simulink model "legacy_torque_controller"  (R2015a)
settings: Solver=ode45  StartTime=0.0  StopTime=10.0  RelTol=1e-3
undefined symbols (not defined in the file): A1_notch_f1, A2_notch_f1, B1_notch_f1, B2_notch_f1, gain_nodes_sea_torque, j_motor, K_notch_f1, k_sea_low, karnopp_model_coulomb_friction, karnopp_model_recursive_filter_sample_number, karnopp_model_static_friction, karnopp_model_velocity_deadzone, kd_sea_percent_of_critical_damping, kp_sea_torque, lateral_motor_efficiency, LEG_MTR_GEAR_RATIO, loaded_unloaded_torque_threshold, max_sagittal_loaded_torque, max_sagittal_unloaded_torque, motor_efficiency_compensation, sample_time, sea_control_torque_cmd_small_threshold
libraries: simulink x4, dsparch4 x1
settings Model: Creator=wmartin  LastModifiedBy=wmartin

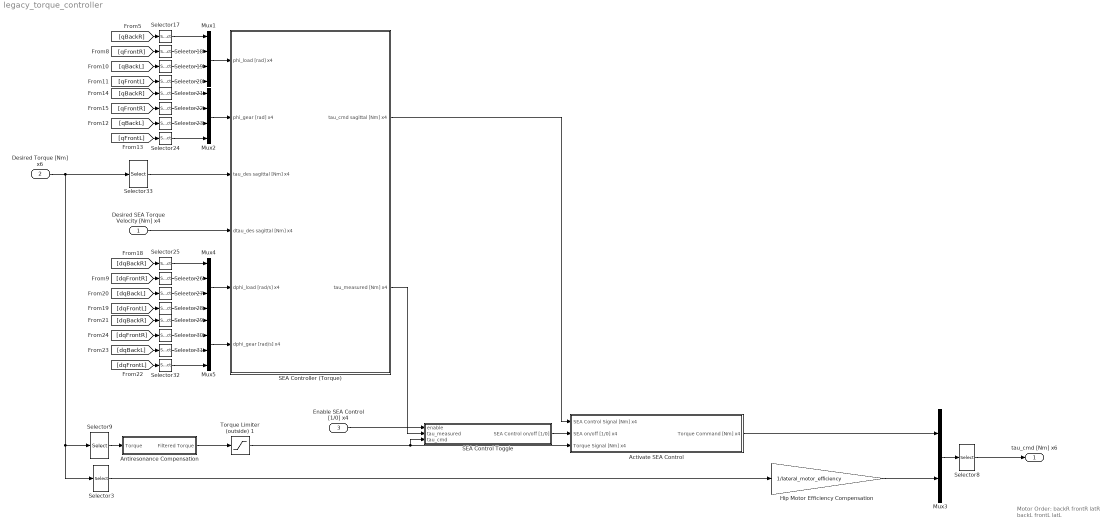
== system legacy_torque_controller ==
  note: Motor Order:
      |
      | backR
      | frontR
      | latR
      | backL
      | frontL
      | latL
  Desired SEA Torque Velocity [Nm] x4 : Inport  OutDataTypeStr=double  PortDimensions=4  SampleTime=sample_time
  Desired Torque [Nm] x6 : Inport  Port=2  OutDataTypeStr=double  PortDimensions=6  SampleTime=sample_time
  Enable SEA Control [1/0] x4 : Inport  Port=3  OutDataTypeStr=boolean  PortDimensions=4  SampleTime=sample_time
  Activate SEA Control : Subsystem
  Antiresonance Compensation : Subsystem
  Hip Motor Efficiency Compensation : Gain  Gain=1/lateral_motor_efficiency
  Mux{1..2,4..5} (4 alike) : Mux
  Mux3 : Mux  Inputs=2
  SEA Control Toggle : Subsystem
  SEA Controller (Torque) : Subsystem
  Selector{17..20,25..28} (8 alike) : Selector  InputPortWidth=2  Indices=[1]
  Selector{21..24,29..32} (8 alike) : Selector  InputPortWidth=2  Indices=[2]
  Selector3 : Selector  InputPortWidth=6  Indices=[3 6]
  Selector33 : Selector  InputPortWidth=6  Indices=[1 2 4 5]
  Selector8 : Selector  InputPortWidth=6  Indices=[1 2 5 3 4 6]
  Selector9 : Selector  InputPortWidth=6  Indices=[1 2 4 5]
  Torque Limiter (outside) 1 : Saturate  UpperLimit=max_sagittal_unloaded_torque  LowerLimit=-max_sagittal_unloaded_torque
      settings: AttributesFormatString=Hi: %<UpperLimit>\nLo: %<LowerLimit>
  tau_cmd [Nm] x6 : Outport  OutDataTypeStr=double  PortDimensions=6  SampleTime=0  InitialOutput=[0 0 0 0 0 0]
  wires:
  Desired Torque [Nm] x6/1 -> Selector9/1, Selector3/1, Selector33/1
  Mux1/1 -> SEA Controller (Torque)/1(phi_load [rad] x4)
  [qBackR] -> Selector17/1
  Selector17/1 -> Mux1/1
  Selector19/1 -> Mux1/3
  Selector18/1 -> Mux1/2
  Selector20/1 -> Mux1/4
  [qFrontR] -> Selector18/1
  [qBackL] -> Selector19/1
  [qFrontL] -> Selector20/1
  Mux2/1 -> SEA Controller (Torque)/2(phi_gear [rad] x4)
  [qBackR] -> Selector21/1
  Selector21/1 -> Mux2/1
  Selector23/1 -> Mux2/3
  Selector22/1 -> Mux2/2
  Selector24/1 -> Mux2/4
  [qFrontR] -> Selector22/1
  [qBackL] -> Selector23/1
  [qFrontL] -> Selector24/1
  Mux4/1 -> SEA Controller (Torque)/5(dphi_load [rad/s] x4)
  [dqBackR] -> Selector25/1
  Selector25/1 -> Mux4/1
  Selector27/1 -> Mux4/3
  Selector26/1 -> Mux4/2
  Selector28/1 -> Mux4/4
  [dqFrontR] -> Selector26/1
  [dqBackL] -> Selector27/1
  [dqFrontL] -> Selector28/1
  Mux5/1 -> SEA Controller (Torque)/6(dphi_gear [rad/s] x4)
  [dqBackR] -> Selector29/1
  Selector29/1 -> Mux5/1
  Selector31/1 -> Mux5/3
  Selector30/1 -> Mux5/2
  Selector32/1 -> Mux5/4
  [dqFrontR] -> Selector30/1
  [dqBackL] -> Selector31/1
  [dqFrontL] -> Selector32/1
  Selector33/1 -> SEA Controller (Torque)/3(tau_des sagittal [Nm] x4)
  Desired SEA Torque Velocity [Nm] x4/1 -> SEA Controller (Torque)/4(dtau_des sagittal [Nm] x4)
  Selector9/1 -> Antiresonance Compensation/1(Torque)
  SEA Controller (Torque)/2(tau_measured [Nm] x4) -> SEA Control Toggle/2(tau_measured)
  Torque Limiter (outside) 1/1 -> SEA Control Toggle/3(tau_cmd), Activate SEA Control/3(Torque Signal [Nm] x4)
  Selector8/1 -> tau_cmd [Nm] x6/1
  Selector3/1 -> Hip Motor Efficiency Compensation/1
  Mux3/1 -> Selector8/1
  Enable SEA Control [1/0] x4/1 -> SEA Control Toggle/1(enable)
  Antiresonance Compensation/1(Filtered Torque) -> Torque Limiter (outside) 1/1
  Activate SEA Control/1(Torque Command [Nm] x4) -> Mux3/1
  Hip Motor Efficiency Compensation/1 -> Mux3/2
  SEA Control Toggle/1(SEA Control on/off [1/0]) -> Activate SEA Control/2("SEA on/off [1/0] x4 ")
  SEA Controller (Torque)/1(tau_cmd sagittal [Nm] x4) -> Activate SEA Control/1(SEA Control Signal [Nm] x4)

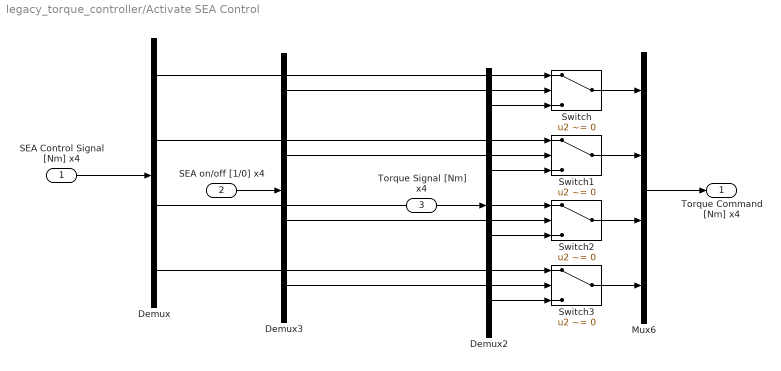
== system legacy_torque_controller/Activate SEA Control ==
  SEA Control Signal [Nm] x4 : Inport
  "SEA on/off [1/0] x4 " : Inport  Port=2
  Torque Signal [Nm] x4 : Inport  Port=3
  Demux : Demux
  Demux2 : Demux
  Demux3 : Demux
  Mux6 : Mux
  Switch{,1..3} (4 alike) : Switch  Criteria=u2 ~= 0
  Torque Command [Nm] x4 : Outport
  wires:
  Torque Signal [Nm] x4/1 -> Demux2/1
  "SEA on/off [1/0] x4 "/1 -> Demux3/1
  SEA Control Signal [Nm] x4/1 -> Demux/1
  Demux2/3 -> Switch2/3
  Demux/2 -> Switch1/1
  Demux3/4 -> Switch3/2
  Demux2/4 -> Switch3/3
  Demux/4 -> Switch3/1
  Switch2/1 -> Mux6/3
  Demux/3 -> Switch2/1
  Demux3/2 -> Switch1/2
  Demux3/3 -> Switch2/2
  Mux6/1 -> Torque Command [Nm] x4/1
  Demux3/1 -> Switch/2
  Switch3/1 -> Mux6/4
  Switch1/1 -> Mux6/2
  Switch/1 -> Mux6/1
  Demux/1 -> Switch/1
  Demux2/1 -> Switch/3
  Demux2/2 -> Switch1/3

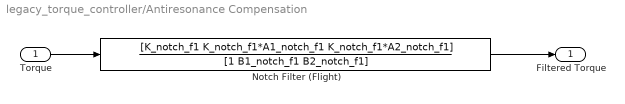
== system legacy_torque_controller/Antiresonance Compensation ==
  Torque : Inport
  Notch Filter (Flight) : DiscreteTransferFcn  Numerator=[K_notch_f1 K_notch_f1*A1_notch_f1 K_notch_f1*A2_notch_f1]  Denominator=[1 B1_notch_f1 B2_notch_f1]  SampleTime=sample_time
  Filtered Torque : Outport
  wires:
  Notch Filter (Flight)/1 -> Filtered Torque/1
  Torque/1 -> Notch Filter (Flight)/1

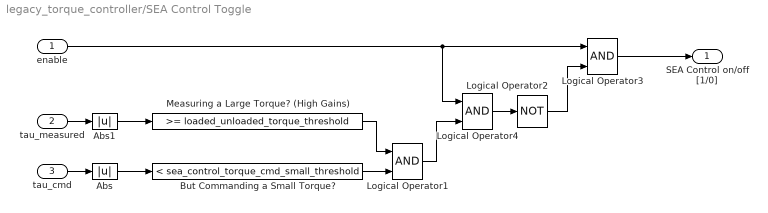
== system legacy_torque_controller/SEA Control Toggle ==
  enable : Inport
  tau_measured : Inport  Port=2
  tau_cmd : Inport  Port=3
  Abs : Abs
  Abs1 : Abs
  But Commanding a Small Torque? : simulink/Logic and Bit Operations/Compare To Constant  relop=<  const=sea_control_torque_cmd_small_threshold  OutDataTypeStr=boolean
  Logical Operator1 : Logic  AllPortsSameDT=off  OutDataTypeStr=boolean
  Logical Operator2 : Logic  Operator=NOT  AllPortsSameDT=off  OutDataTypeStr=boolean
  Logical Operator3 : Logic  AllPortsSameDT=off  OutDataTypeStr=boolean
  Logical Operator4 : Logic  AllPortsSameDT=off  OutDataTypeStr=boolean
  Measuring a Large Torque? (High Gains) : simulink/Logic and Bit Operations/Compare To Constant  relop=>=  const=loaded_unloaded_torque_threshold  OutDataTypeStr=boolean
  SEA Control on/off [1/0] : Outport
  wires:
  Measuring a Large Torque? (High Gains)/1 -> Logical Operator1/1
  enable/1 -> Logical Operator3/1, Logical Operator4/1
  Logical Operator4/1 -> Logical Operator2/1
  Logical Operator2/1 -> Logical Operator3/2
  Logical Operator3/1 -> SEA Control on/off [1/0]/1
  Abs1/1 -> Measuring a Large Torque? (High Gains)/1
  tau_measured/1 -> Abs1/1
  Abs/1 -> But Commanding a Small Torque?/1
  tau_cmd/1 -> Abs/1
  Logical Operator1/1 -> Logical Operator4/2
  But Commanding a Small Torque?/1 -> Logical Operator1/2

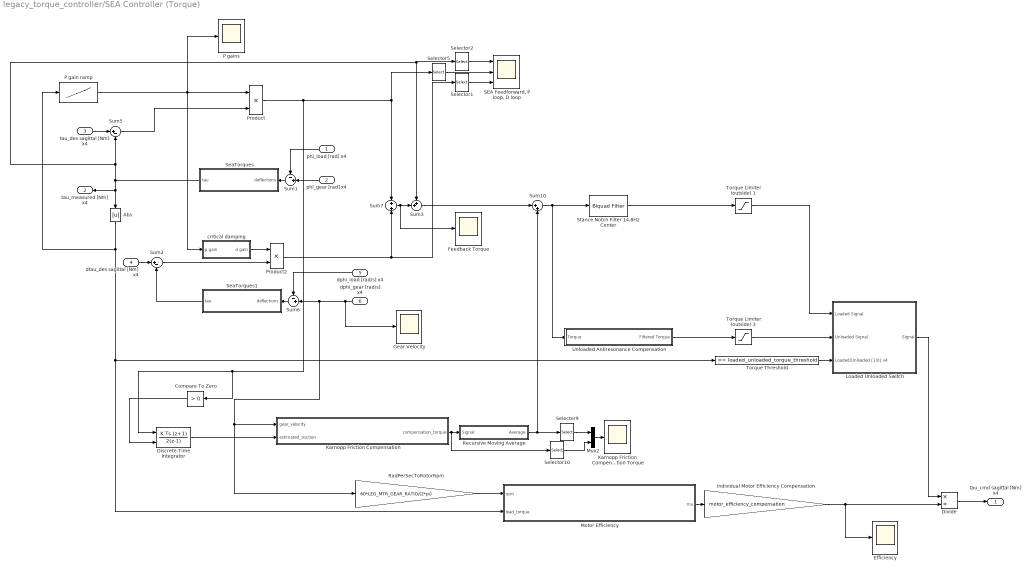
== system legacy_torque_controller/SEA Controller (Torque) ==
  phi_load [rad] x4 : Inport
  phi_gear [rad] x4 : Inport  Port=2
  tau_des sagittal [Nm] x4 : Inport  Port=3
  dtau_des sagittal [Nm] x4 : Inport  Port=4
  dphi_load [rad/s] x4 : Inport  Port=5
  dphi_gear [rad/s] x4 : Inport  Port=6
  Abs : Abs
  Compare To Zero : simulink/Logic and Bit Operations/Compare To Zero  relop=>  OutDataTypeStr=boolean
  Discrete-Time Integrator : DiscreteIntegrator  IntegratorMethod=Integration: Trapezoidal  gainval=karnopp_model_integration_constant  ExternalReset=either  InitialConditionSetting=State (most efficient)  SampleTime=sample_time  LimitOutput=on  UpperSaturationLimit=karnopp_model_static_friction  LowerSaturationLimit=-karnopp_model_static_friction
  Divide : Product  Inputs=*/
  Efficiency : Scope
      settings: YMin=0.45  YMax=0.775  SaveName=ScopeData4  SampleInput=on
  Feedback Torque : Scope
      settings: YMin=-150  YMax=125  SaveName=ScopeData9  SampleInput=on
  Gear Velocity : Scope
      settings: YMin=-0.25  YMax=0.3  SaveName=ScopeData8  SampleInput=on
  Individual Motor Efficiency Compensation : Gain  Gain=motor_efficiency_compensation
  Karnopp Friction Compensation : MATLAB Function  TreatAsAtomicUnit=on
  Karnopp Friction Compensation Torque : Scope
      settings: YMin=-40  YMax=40  SaveName=ScopeData10  SampleInput=on
  Loaded Unloaded Switch : Subsystem
  Motor Efficiency : MATLAB Function  TreatAsAtomicUnit=on
  Mux2 : Mux  Inputs=2
  P gain ramp : Lookup_n-D  NumberOfTableDimensions=1  BreakpointsForDimension1=gain_nodes_sea_torque  Table=kp_sea_torque  InternalRulePriority=Speed  RndMeth=Simplest  InputSameDT=on
  P gains : Scope
      settings: YMin=0.1  YMax=2.3  SaveName=ScopeData6  SampleInput=on
  Product : Product  SampleTime=sample_time  RndMeth=Zero
  Product2 : Product  RndMeth=Zero
  RadPerSecToRotorRpm : Gain  Gain=60*LEG_MTR_GEAR_RATIO/(2*pi)
  Recursive Moving Average : Subsystem
  "SEA Feedforward, P loop, D loop" : Scope  NumInputPorts=3
      settings: YMin=-200~-80~-30  YMax=250~70~25  SaveName=ScopeData3  SampleInput=on
  SeaTorques : MATLAB Function  TreatAsAtomicUnit=on
  SeaTorques1 : MATLAB Function  TreatAsAtomicUnit=on
  Selector{1..2,5,9..10} (5 alike) : Selector  InputPortWidth=4  Indices=[1 2]
  Stance Notch Filter 14.8Hz Center : dsparch4/Biquad Filter  Tag=BlockMethodSubSystem  IIRFiltStruct=Direct form II  CoeffSource=Specify via dialog  BiQuadCoeffs=[1.0043405224042976 -2 1.0043376322156812 1 -1.9864973201238227 0.99417420144306112;1.0043409871477107 -1.9999999999999998 1.004338097267472 1 -1.9837994373655783 0.99346561709978676;1.0043421997869275 -2 1.0043364197180722 1 -1.9790895333620613 0.98767741587524949]  a0Flag=Warning  IC=0  ICnum=0  ICden=0  InputProcessing=Columns as channels (frame based)  denAccumFracLength=30  denProdOutputFracLength=30  secondMemoryFracLength=15  roundingMode=Floor  overflowMode=off  ScaleValues=[0.00051103132043923321;1;1;1907.7713598660641]  optimizeScaleValues=on  ScaleValueMode=Specify via input port (g)  scaleValueFracLength=14  FilterSource=Specify via dialog  FilterObject=Hm_biquad
  Sum1 : Sum  Inputs=-+|
  Sum10 : Sum  Inputs=|++
  Sum2 : Sum  Inputs=|+-
  Sum3 : Sum  Inputs=++|
  Sum5 : Sum  Inputs=|+-
  Sum6 : Sum  Inputs=-+|
  Sum7 : Sum  Inputs=+|+
  Torque Limiter (outside) 1 : Saturate  UpperLimit=max_sagittal_loaded_torque  LowerLimit=-max_sagittal_loaded_torque
      settings: AttributesFormatString=Hi: %<UpperLimit>\nLo: %<LowerLimit>
  Torque Limiter (outside) 3 : Saturate  UpperLimit=max_sagittal_unloaded_torque  LowerLimit=-max_sagittal_unloaded_torque
      settings: AttributesFormatString=Hi: %<UpperLimit>\nLo: %<LowerLimit>
  Torque Threshold : simulink/Logic and Bit Operations/Compare To Constant  relop=>=  const=loaded_unloaded_torque_threshold  OutDataTypeStr=boolean
  Unloaded Antiresonance Compensation : Subsystem
  critical damping : Subsystem
  tau_cmd sagittal [Nm] x4 : Outport
  tau_measured [Nm] x4 : Outport  Port=2
  wires:
  Selector10/1 -> Mux2/2
  Mux2/1 -> Karnopp Friction Compensation Torque/1
  Recursive Moving Average/1(Average) -> Sum10/2, Selector9/1
  Selector9/1 -> Mux2/1
  Compare To Zero/1 -> Discrete-Time Integrator/2
  Product/1 -> Sum7/1, Selector5/1, Discrete-Time Integrator/1, Compare To Zero/1
  Discrete-Time Integrator/1 -> Karnopp Friction Compensation/2(estimated_stiction)
  dphi_gear [rad/s] x4/1 -> Gear Velocity/1, RadPerSecToRotorRpm/1, Karnopp Friction Compensation/1(gear_velocity), Sum6/2
  Sum10/1 -> Stance Notch Filter 14.8Hz Center/1, Unloaded Antiresonance Compensation/1(Torque)
  Karnopp Friction Compensation/1(compensation_torque) -> Recursive Moving Average/1(Signal), Selector10/1
  Sum7/1 -> Sum3/2, Feedback Torque/1
  dphi_load [rad/s] x4/1 -> Sum6/1
  Selector2/1 -> "SEA Feedforward, P loop, D loop"/1
  Selector5/1 -> "SEA Feedforward, P loop, D loop"/2
  Selector1/1 -> "SEA Feedforward, P loop, D loop"/3
  Divide/1 -> tau_cmd sagittal [Nm] x4/1
  dtau_des sagittal [Nm] x4/1 -> Sum2/1
  Stance Notch Filter 14.8Hz Center/1 -> Torque Limiter (outside) 1/1
  Individual Motor Efficiency Compensation/1 -> Efficiency/1, Divide/2
  Sum1/1 -> SeaTorques/1(deflections)
  SeaTorques/1(tau) -> Sum5/2, Selector2/1, Sum3/1, tau_measured [Nm] x4/1, Abs/1
  Motor Efficiency/1(mu) -> Individual Motor Efficiency Compensation/1
  RadPerSecToRotorRpm/1 -> Motor Efficiency/1(rpm)
  Loaded Unloaded Switch/1(Signal) -> Divide/1
  Abs/1 -> Torque Threshold/1, Motor Efficiency/2(load_torque), P gain ramp/1
  Sum3/1 -> Sum10/1
  Unloaded Antiresonance Compensation/1(Filtered Torque) -> Torque Limiter (outside) 3/1
  critical damping/1(d gain) -> Product2/1
  Torque Threshold/1 -> Loaded Unloaded Switch/3(Loaded/Unloaded [1/0] x4)
  Torque Limiter (outside) 3/1 -> Loaded Unloaded Switch/2(Unloaded Signal)
  Torque Limiter (outside) 1/1 -> Loaded Unloaded Switch/1(Loaded Signal)
  P gain ramp/1 -> Product/1, critical damping/1(p gain), P gains/1
  phi_load [rad] x4/1 -> Sum1/1
  phi_gear [rad] x4/1 -> Sum1/2
  tau_des sagittal [Nm] x4/1 -> Sum5/1
  Sum6/1 -> SeaTorques1/1(deflections)
  SeaTorques1/1(tau) -> Sum2/2
  Sum5/1 -> Product/2
  Sum2/1 -> Product2/2
  Product2/1 -> Sum7/2, Selector1/1

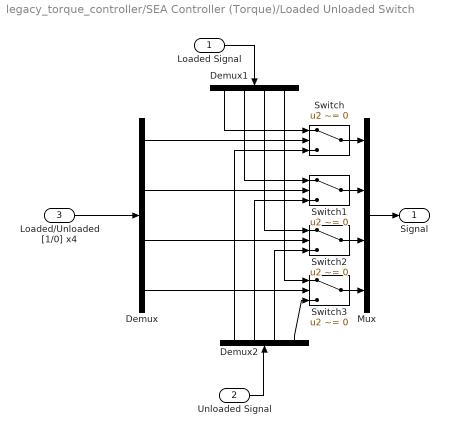
== system legacy_torque_controller/SEA Controller (Torque)/Loaded Unloaded Switch ==
  Loaded Signal : Inport
  Unloaded Signal : Inport  Port=2
  Loaded/Unloaded [1/0] x4 : Inport  Port=3
  Demux : Demux
  Demux1 : Demux
  Demux2 : Demux
  Mux : Mux
  Switch{,1..3} (4 alike) : Switch  Criteria=u2 ~= 0
  Signal : Outport
  wires:
  Demux/4 -> Switch3/2
  Demux/3 -> Switch2/2
  Demux/2 -> Switch1/2
  Switch1/1 -> Mux/2
  Switch2/1 -> Mux/3
  Switch3/1 -> Mux/4
  Loaded/Unloaded [1/0] x4/1 -> Demux/1
  Mux/1 -> Signal/1
  Switch/1 -> Mux/1
  Demux/1 -> Switch/2
  Loaded Signal/1 -> Demux1/1
  Demux1/1 -> Switch/1
  Demux1/2 -> Switch1/1
  Demux1/3 -> Switch2/1
  Demux1/4 -> Switch3/1
  Unloaded Signal/1 -> Demux2/1
  Demux2/4 -> Switch3/3
  Demux2/3 -> Switch2/3
  Demux2/2 -> Switch1/3
  Demux2/1 -> Switch/3

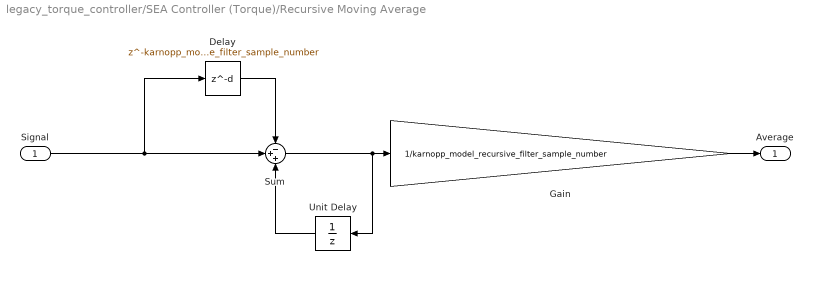
== system legacy_torque_controller/SEA Controller (Torque)/Recursive Moving Average ==
  Signal : Inport
  Delay : Delay  DelayLength=karnopp_model_recursive_filter_sample_number  InitialCondition=0  UseCircularBuffer=on  SampleTime=sample_time
  Gain : Gain  Gain=1/karnopp_model_recursive_filter_sample_number
  Sum : Sum  Inputs=-++
  Unit Delay : UnitDelay  SampleTime=sample_time
  Average : Outport
  wires:
  Signal/1 -> Delay/1, Sum/2
  Sum/1 -> Gain/1, Unit Delay/1
  Delay/1 -> Sum/1
  Gain/1 -> Average/1
  Unit Delay/1 -> Sum/3

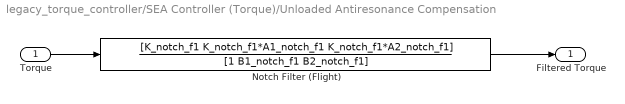
== system legacy_torque_controller/SEA Controller (Torque)/Unloaded Antiresonance Compensation ==
  Torque : Inport
  Notch Filter (Flight) : DiscreteTransferFcn  Numerator=[K_notch_f1 K_notch_f1*A1_notch_f1 K_notch_f1*A2_notch_f1]  Denominator=[1 B1_notch_f1 B2_notch_f1]  SampleTime=sample_time
  Filtered Torque : Outport
  wires:
  Torque/1 -> Notch Filter (Flight)/1
  Notch Filter (Flight)/1 -> Filtered Torque/1

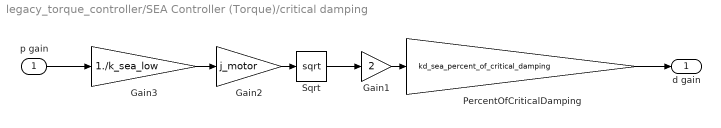
== system legacy_torque_controller/SEA Controller (Torque)/critical damping ==
  p gain : Inport
  Gain1 : Gain  Gain=2
  Gain2 : Gain  Gain=j_motor
  Gain3 : Gain  Gain=1./k_sea_low
  PercentOfCriticalDamping : Gain  Gain=kd_sea_percent_of_critical_damping
  Sqrt : Sqrt  SaturateOnIntegerOverflow=on
  d gain : Outport
  wires:
  PercentOfCriticalDamping/1 -> d gain/1
  Gain1/1 -> PercentOfCriticalDamping/1
  Gain3/1 -> Gain2/1
  Gain2/1 -> Sqrt/1
  Sqrt/1 -> Gain1/1
  p gain/1 -> Gain3/1

== matlab function legacy_torque_controller/SEA Controller (Torque)/SeaTorques1 ==
  data: deflections input; tau output
function tau = SeaSpringForce(deflections)
    tau = SeaSpringForce(deflections);
end

== matlab function legacy_torque_controller/SEA Controller (Torque)/Karnopp Friction Compensation ==
  data: gear_velocity input; estimated_stiction input; compensation_torque output; karnopp_model_velocity_deadzone parameter; karnopp_model_coulomb_friction parameter; karnopp_model_static_friction parameter
% Compensate for stiction and coulomb friction using the Karnopp model
% Assumes velocity is small in the "dead zone"
function compensation_torque = friction_compensation(gear_velocity, estimated_stiction, karnopp_model_velocity_deadzone, karnopp_model_coulomb_friction, karnopp_model_static_friction)
    
    % Coulomb compensation at high velocities
    compensation_torque = karnopp_model_coulomb_friction.*sign(gear_velocity);
    
    % Stiction compensation inside velocity deadzone
    inside_deadzone = abs(gear_velocity) <= karnopp_model_velocity_deadzone;
    compensation_torque(inside_deadzone) = estimated_stiction(inside_deadzone);
    
end

== matlab function legacy_torque_controller/SEA Controller (Torque)/SeaTorques ==
  data: deflections input; tau output
function tau = SeaSpringForce(deflections)
    tau = SeaSpringForce(deflections);
end

== matlab function legacy_torque_controller/SEA Controller (Torque)/Motor Efficiency ==
  data: rpm input; mu output; load_torque input
function mu = HarmonicDriveEfficiency(rpm, load_torque)
    mu = HarmonicDriveEfficiency(rpm, load_torque);
end
